simulink model "BF1"  (R2021b)
settings: Solver=VariableStepAuto  StartTime=0.0  StopTime=10.0  RelTol=1e-3
values from neighbouring files (symbols this model uses):
  plant = ss(a,b,c,d)    [demarrage.m]
undefined symbols (not defined in the file or in its folder): H, Ky
settings Model: Creator=driss  LastModifiedBy=driss
settings DebuggingCC: AlgebraicLoopMsg=none

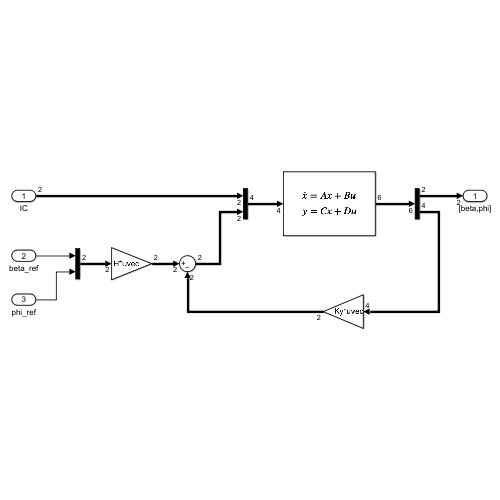
[thumbnail: Simulink's stored preview of the top-level diagram]
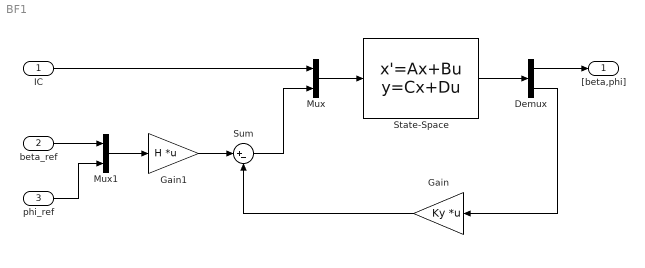
== system BF1 ==
  IC : Inport
  beta_ref : Inport  Port=2
  phi_ref : Inport  Port=3
  Demux : Demux  Outputs=[2 4]
  Gain : Gain  Gain=Ky  Multiplication=Matrix(K*u) (u vector)
  Gain1 : Gain  Gain=H  Multiplication=Matrix(K*u) (u vector)
  Mux : Mux  Inputs=[2 2]
  Mux1 : Mux  Inputs=[1 1]
  State-Space : StateSpace  A=plant.A  B=[[1 0; 0 0; 0 0 ;0 1] plant.B]  C=[1 0 0 0; 0 0 0 1;plant.C]  D=[zeros(6,2) [zeros(2); plant.D]]  InitialCondition=0
  Sum : Sum  Inputs=|+-
  "[beta,phi]" : Outport
  wires:
  Demux/2 -> Gain/1
  Demux/1 -> "[beta,phi]"/1
  State-Space/1 -> Demux/1
  Mux/1 -> State-Space/1
  IC/1 -> Mux/1
  Gain/1 -> Sum/2
  Sum/1 -> Mux/2
  beta_ref/1 -> Mux1/1
  phi_ref/1 -> Mux1/2
  Gain1/1 -> Sum/1
  Mux1/1 -> Gain1/1
